simulink model "VehicleModel"  (R2015b)
settings: Solver=VariableStepAuto  StartTime=0.0  StopTime=10.0  RelTol=1e-3
undefined symbols (not defined in the file): Gamma, v
settings Model: Creator=GianAndrea  LastModifiedBy=GianAndrea

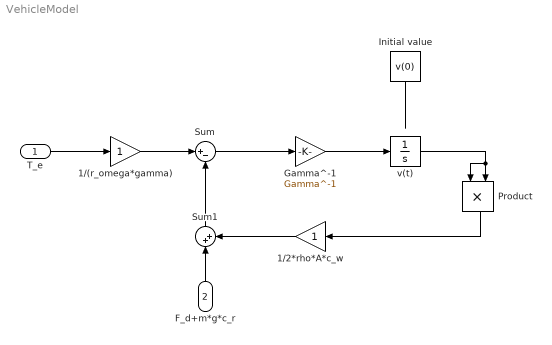
== system VehicleModel ==
  T_e : Inport
  F_d+m*g*c_r : Inport  Port=2
  1/(r_omega*gamma) : Gain
  1/2*rho*A*c_w : Gain
  Gamma^-1 : Gain  Gain=Gamma^-1
  Initial value : Constant  Value=v(0)
  Product : Product
  Sum : Sum  Inputs=|+-
  Sum1 : Sum  Inputs=|++
  v(t) : Integrator
  wires:
  Initial value/1 -> ?
  Sum1/1 -> Sum/2
  1/2*rho*A*c_w/1 -> Sum1/2
  v(t)/1 -> Product/1, Product/2
  Product/1 -> 1/2*rho*A*c_w/1
  Gamma^-1/1 -> v(t)/1
  Sum/1 -> Gamma^-1/1
  1/(r_omega*gamma)/1 -> Sum/1
  T_e/1 -> 1/(r_omega*gamma)/1
  F_d+m*g*c_r/1 -> Sum1/1
